simulink model "ibob_phased_array_2k"  (Simulink 7.1)
settings: Solver=ode45  StartTime=0.0  StopTime=70  RelTol=1e-3
undefined symbols (not defined in the file or in its folder): iBOB
libraries: xbsIndex_r4 x1407, xps_library x46, cfa_library x16, casper_library_sources x8, casper_library_misc x4
(part 1 of 18)
settings Model: Creator=Administrator  LastModifiedBy=Rurik A Primiani
settings DebuggingCC: SaveWithParameterizedLinksMsg=none  SignalResolutionControl=TryResolveAllWithWarning  MultiTaskDSMMsg=warning  MultiTaskCondExecSysMsg=none  StrictBusMsg=None
settings RTWCC: IncludeERTFirstTime=on
settings GRTTargetCC: TargetFcnLib=ansi_tfl_tmw.mat

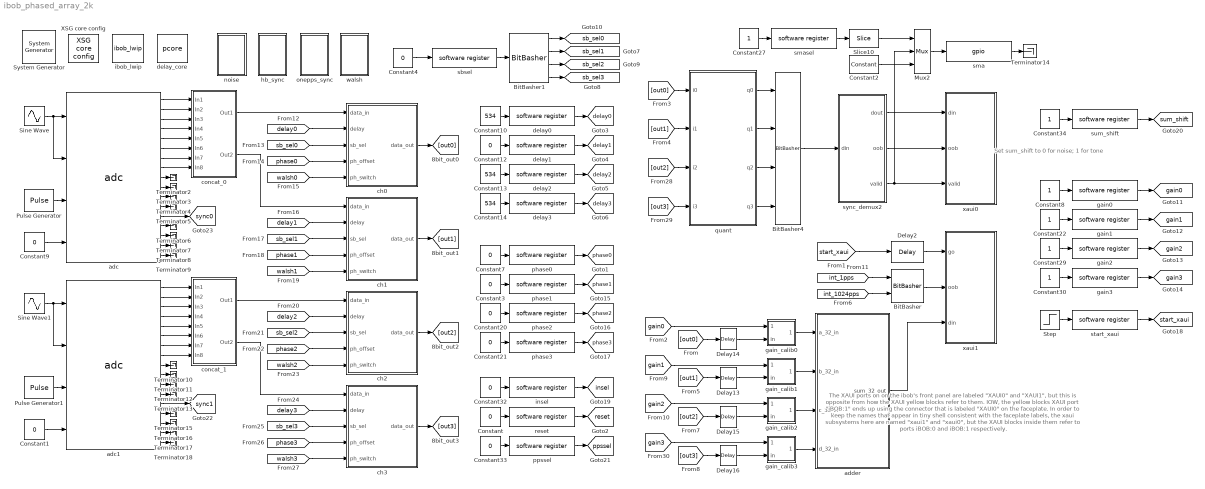
== system ibob_phased_array_2k ==
  note: The XAUI ports on on the ibob's front panel are labeled "XAUI0"
      | and "XAUI1", but this is opposite from how the XAUI yellow blocks
      | refer to them.  IOW, the yellow blocks XAUI port "iBOB:1" ends up
      | using the connector that is labeled "XAUI0" on the faceplate.
      |
      | In order to keep the names that appear in tiny shell consistent with
      | the faceplate labels, the xaui subsystems here are named "xaui1"
      | and "xaui0", but the XAUI blocks inside them refer to ports iBOB:0
      | and iBOB:1 respectively.
  note: Set sum_shift to 0 for noise; 1 for tone
  " System Generator" : xbsIndex_r4/ System Generator  Tag=genX  SystemSampleTime=-1  xilinxfamily=virtex2p  part=xc2vp50  speed=-7  package=ff1152  synthesis_tool=XST  clock_wrapper=Clock Enables  directory=./ibob_phased_array_2k/sysgen  testbench=off  simulink_period=1  sysclk_period=3.9063  dcm_input_clock_period=100  incr_netlist=off  trim_vbits=Everywhere in SubSystem  dbl_ovrd=According to Block Masks  core_generation=According to Block Masks  run_coregen=off  deprecated_control=off  eval_field=0  block_type=sysgen
      settings: block_version=10.1.3
  BitBasher : xbsIndex_r4/BitBasher  bitexpr=|  display_expr=off  sr_1=1  arith_type1=Unsigned  bin_pt1=0  sr_2=2  arith_type2=Unsigned  bin_pt2=0  sr_3=3  arith_type3=Unsigned  bin_pt3=0  sr_4=4  arith_type4=Unsigned  bin_pt4=0  dbl_ovrd=off  block_type=bitbasher
      | <html><head><meta name="qrichtext" content="1" /><style type="text/css">
      | p, li { white-space: pre-wrap; }
      | </style></head><body style=" font-family:'MS Shell Dlg 2'; font-size:8.25pt; font-weight:400; font-style:normal;">
      | <p style=" margin-top:12px; margin-bottom:12px; margin-left:0px; margin-right:0px; -qt-block-indent:0; text-indent:0px; font-family:'MS Shell Dlg'; font-size:8pt;">oob={2'b00,pps1,pps1024}</p></body></html>
      settings: block_version=10.1.3
  BitBasher1 : xbsIndex_r4/BitBasher  bitexpr=|  display_expr=off  sr_1=1  arith_type1=Unsigned  bin_pt1=0  sr_2=2  arith_type2=Unsigned  bin_pt2=0  sr_3=3  arith_type3=Unsigned  bin_pt3=0  sr_4=4  arith_type4=Unsigned  bin_pt4=0  dbl_ovrd=off  block_type=bitbasher
      | <html><head><meta name="qrichtext" content="1" /><style type="text/css">
      | p, li { white-space: pre-wrap; }
      | </style></head><body style=" font-family:'MS Shell Dlg 2'; font-size:8.25pt; font-weight:400; font-style:normal;">
      | <p style=" margin-top:12px; margin-bottom:12px; margin-left:0px; margin-right:0px; -qt-block-indent:0; text-indent:0px; font-family:'MS Shell Dlg'; font-size:8pt;">sel0={sel[0]}<br />sel1={sel[4]}<br />sel2={sel[8]}<br />sel3={sel[12]}<br /></p></body></html>
      settings: block_version=10.1.3
  BitBasher4 : xbsIndex_r4/BitBasher  bitexpr=|  display_expr=off  sr_1=1  arith_type1=Unsigned  bin_pt1=0  sr_2=2  arith_type2="Signed  (2's comp)"  bin_pt2=7  sr_3=3  arith_type3="Signed  (2's comp)"  bin_pt3=7  sr_4=4  arith_type4="Signed  (2's comp)"  bin_pt4=7  dbl_ovrd=off  block_type=bitbasher
      | <html><head><meta name="qrichtext" content="1" /><style type="text/css">
      | p, li { white-space: pre-wrap; }
      | </style></head><body style=" font-family:'MS Shell Dlg 2'; font-size:8.25pt; font-weight:400; font-style:normal;">
      | <p style=" margin-top:0px; margin-bottom:0px; margin-left:0px; margin-right:0px; -qt-block-indent:0; text-indent:0px; font-size:8pt;">out={in0,in1,in2,in3}</p></body></html>
      settings: block_version=10.1.3
  Constant{,1,3..4,7,9,12,20..21,32..33} (11 alike) : Constant  Value=0  OutDataType=sfix(16)  OutScaling=2^0
  Constant10 : Constant  Value=534  OutDataType=sfix(16)  OutScaling=2^0
  Constant13 : Constant  Value=534  OutDataType=sfix(16)  OutScaling=2^0
  Constant14 : Constant  Value=534  OutDataType=sfix(16)  OutScaling=2^0
  Constant2 : xbsIndex_r4/Constant  arith_type=Boolean  const=0  n_bits=16  bin_pt=14  explicit_period=off  period=1  equ=P=C  opselect=C  inp2=PCIN>>17  opr=+  inp1=P  carry=CIN  dbl_ovrd=off  block_type=constant
  Constant{8,22,27,29..30,34} (6 alike) : Constant  OutDataType=sfix(16)  OutScaling=2^0
  Delay{2,13..16} (5 alike) : xbsIndex_r4/Delay  en=off  latency=10  dbl_ovrd=off  reg_retiming=on  block_type=delay
      settings: xl_area=[0, 0, 0, 0, 0, 0, 0]
  Mux2 : xbsIndex_r4/Mux  inputs=2  en=off  latency=2  precision=Full  arith_type="Signed  (2's comp)"  n_bits=8  bin_pt=2  quantization=Truncate  overflow=Wrap  dbl_ovrd=off  block_type=mux
      settings: xl_area=[0, 0, 0, 0, 0, 0, 0]
  Pulse Generator : DiscretePulseGenerator  Period=100  PulseWidth=20
  Pulse Generator1 : DiscretePulseGenerator  Period=100  PulseWidth=20
  Sine Wave : Sin  SineType=Sample based  Amplitude=0.9  Frequency=6.4340e+9  Samples=60  SampleTime=1/4
  Sine Wave1 : Sin  SineType=Sample based  Amplitude=0.9  Frequency=6.4340e+9  Samples=60  SampleTime=1/4
  Slice10 : xbsIndex_r4/Slice  nbits=1  boolean_output=off  mode=Lower Bit Location + Width  bit1=0  base1=MSB of Input  bit0=0  base0=LSB of Input  dbl_ovrd=off  block_type=slice
      settings: infoedit="Extracts a given range of bits from each input sample and presents it at the output.  The output type is ordinarily unsigned with binary point at zero, but can be Boolean when the slice is one bit wide.<P><P>Hardware notes: In hardware this block costs nothing."  block_version=10.1.3
  Step : Step  Time=100  SampleTime=0
  Terminator{2..18} (17 alike) : Terminator
  XSG core config : xps_library/XSG core config  Tag=xps:xsg  SystemSampleTime=-1  hw_sys=iBOB  ibob_linux=off  clk_src=adc0_clk  iBOB_clk_src=adc0_clk  BEE2_ctrl_clk_src=sys_clk  BEE2_usr_clk_src=sys_clk  ROACH_clk_src=sys_clk  CORR_clk_src=sys_clk  gpio_clk_io_group=iBOB:sma  gpio_clk_bit_index=0  clk_rate=256  sample_period=1  synthesis_tool=XST  mpc_type=powerpc405
  adc : xps_library/adc  Tag=xps:adc  SystemSampleTime=-1  adc_brd=adc0  adc_clk_rate=1024  adc_interleave=off  sample_period=1
  adc1 : xps_library/adc  Tag=xps:adc  SystemSampleTime=-1  adc_brd=adc1  adc_clk_rate=1024  adc_interleave=off  sample_period=1
  adder : Subsystem
  ch0 : Subsystem
  ch1 : Subsystem
  ch2 : Subsystem
  ch3 : Subsystem
  concat_0 : Subsystem
  concat_1 : Subsystem
  delay0 : xps_library/software register  Tag=xps:sw_reg  SystemSampleTime=-1  io_dir=From Processor  arith_type=Unsigned  bitwidth=32  bin_pt=0  sample_period=1  gw_name=ibob_phased_array_2k_delay0_user_data_out
      link override ibob_phased_array_2k_delay0_user_data_out: arith_type=Unsigned  n_bits=32  bin_pt=0  period=1
      link override ibob_phased_array_2k_delay1_user_data_out: arith_type=Unsigned  n_bits=32  bin_pt=0  period=1
  delay1 : xps_library/software register  Tag=xps:sw_reg  SystemSampleTime=-1  io_dir=From Processor  arith_type=Unsigned  bitwidth=32  bin_pt=0  sample_period=1  gw_name=ibob_phased_array_2k_delay1_user_data_out
      link override ibob_phased_array_2k_delay1_user_data_out: arith_type=Unsigned  n_bits=32  bin_pt=0  period=1
      link override ibob_phased_array_2k_delay2_user_data_out: arith_type=Unsigned  n_bits=32  bin_pt=0  period=1
  delay2 : xps_library/software register  Tag=xps:sw_reg  SystemSampleTime=-1  io_dir=From Processor  arith_type=Unsigned  bitwidth=32  bin_pt=0  sample_period=1  gw_name=ibob_phased_array_2k_delay2_user_data_out
      link override ibob_phased_array_2k_delay2_user_data_out: arith_type=Unsigned  n_bits=32  bin_pt=0  period=1
      link override ibob_phased_array_2k_delay3_user_data_out: arith_type=Unsigned  n_bits=32  bin_pt=0  period=1
  delay3 : xps_library/software register  Tag=xps:sw_reg  SystemSampleTime=-1  io_dir=From Processor  arith_type=Unsigned  bitwidth=32  bin_pt=0  sample_period=1  gw_name=ibob_phased_array_2k_delay3_user_data_out
      link override ibob_phased_array_2k_delay3_user_data_out: arith_type=Unsigned  n_bits=32  bin_pt=0  period=1
      link override ibob_phased_array_2k_delay4_user_data_out: arith_type=Unsigned  n_bits=32  bin_pt=0  period=1
  delay_core : xps_library/pcore  Tag=xps:pcore  SystemSampleTime=-1  pcore_path=delay_core/delay_core.ngc
  gain0 : xps_library/software register  Tag=xps:sw_reg  SystemSampleTime=-1  io_dir=From Processor  arith_type=Unsigned  bitwidth=32  bin_pt=0  sample_period=1  gw_name=ibob_phased_array_2k_gain0_user_data_out
      link override ibob_phased_array_2k_gain0_user_data_out: arith_type=Unsigned  n_bits=32  bin_pt=0  period=1
  gain1 : xps_library/software register  Tag=xps:sw_reg  SystemSampleTime=-1  io_dir=From Processor  arith_type=Unsigned  bitwidth=32  bin_pt=0  sample_period=1  gw_name=ibob_phased_array_2k_gain1_user_data_out
      link override ibob_phased_array_2k_gain1_user_data_out: arith_type=Unsigned  n_bits=32  bin_pt=0  period=1
  gain2 : xps_library/software register  Tag=xps:sw_reg  SystemSampleTime=-1  io_dir=From Processor  arith_type=Unsigned  bitwidth=32  bin_pt=0  sample_period=1  gw_name=ibob_phased_array_2k_gain2_user_data_out
      link override ibob_phased_array_2k_gain2_user_data_out: arith_type=Unsigned  n_bits=32  bin_pt=0  period=1
  gain3 : xps_library/software register  Tag=xps:sw_reg  SystemSampleTime=-1  io_dir=From Processor  arith_type=Unsigned  bitwidth=32  bin_pt=0  sample_period=1  gw_name=ibob_phased_array_2k_gain3_user_data_out
      link override ibob_phased_array_2k_gain3_user_data_out: arith_type=Unsigned  n_bits=32  bin_pt=0  period=1
  gain_calib0 : Subsystem
  gain_calib1 : Subsystem
  gain_calib2 : Subsystem
  gain_calib3 : Subsystem
  hb_sync : Subsystem
  ibob_lwip : xps_library/ibob_lwip  SystemSampleTime=-1
      link override macbits/convert: arith_type=Unsigned  n_bits=32  bin_pt=0
      link override machdr/ibob_phased_array_2k_ibob_lwip_machdr_gateway: arith_type=Unsigned  n_bits=20  bin_pt=0  period=sample_period
  insel : xps_library/software register  Tag=xps:sw_reg  SystemSampleTime=-1  io_dir=From Processor  arith_type=Unsigned  bitwidth=32  bin_pt=0  sample_period=1  gw_name=ibob_phased_array_2k_insel_user_data_out
      link override ibob_phased_array_2k_insel_user_data_out: arith_type=Unsigned  n_bits=32  bin_pt=0  period=1
      link override ibob_phased_array_2k_reset_user_data_out: arith_type=Unsigned  n_bits=32  bin_pt=0  period=1
  noise : Subsystem
  onepps_sync : Subsystem
  phase0 : xps_library/software register  Tag=xps:sw_reg  SystemSampleTime=-1  io_dir=From Processor  arith_type=Unsigned  bitwidth=32  bin_pt=0  sample_period=1  gw_name=ibob_phased_array_2k_phase0_user_data_out
      link override ibob_phased_array_2k_bypass1_user_data_out: arith_type=Unsigned  n_bits=32  bin_pt=0  period=1
      link override ibob_phased_array_2k_phase0_user_data_out: arith_type=Unsigned  n_bits=32  bin_pt=0  period=1
  phase1 : xps_library/software register  Tag=xps:sw_reg  SystemSampleTime=-1  io_dir=From Processor  arith_type=Unsigned  bitwidth=32  bin_pt=0  sample_period=1  gw_name=ibob_phased_array_2k_phase1_user_data_out
      link override ibob_phased_array_2k_bypass2_user_data_out: arith_type=Unsigned  n_bits=32  bin_pt=0  period=1
      link override ibob_phased_array_2k_phase1_user_data_out: arith_type=Unsigned  n_bits=32  bin_pt=0  period=1
  phase2 : xps_library/software register  Tag=xps:sw_reg  SystemSampleTime=-1  io_dir=From Processor  arith_type=Unsigned  bitwidth=32  bin_pt=0  sample_period=1  gw_name=ibob_phased_array_2k_phase2_user_data_out
      link override ibob_phased_array_2k_bypass3_user_data_out: arith_type=Unsigned  n_bits=32  bin_pt=0  period=1
      link override ibob_phased_array_2k_phase2_user_data_out: arith_type=Unsigned  n_bits=32  bin_pt=0  period=1
  phase3 : xps_library/software register  Tag=xps:sw_reg  SystemSampleTime=-1  io_dir=From Processor  arith_type=Unsigned  bitwidth=32  bin_pt=0  sample_period=1  gw_name=ibob_phased_array_2k_phase3_user_data_out
      link override ibob_phased_array_2k_bypass4_user_data_out: arith_type=Unsigned  n_bits=32  bin_pt=0  period=1
      link override ibob_phased_array_2k_phase3_user_data_out: arith_type=Unsigned  n_bits=32  bin_pt=0  period=1
  ppssel : xps_library/software register  Tag=xps:sw_reg  SystemSampleTime=-1  io_dir=From Processor  arith_type=Unsigned  bitwidth=32  bin_pt=0  sample_period=1  gw_name=ibob_phased_array_2k_ppssel_user_data_out
      link override ibob_phased_array_2k_ppssel_user_data_out: arith_type=Unsigned  n_bits=32  bin_pt=0  period=1
      link override ibob_phased_array_2k_reset_user_data_out: arith_type=Unsigned  n_bits=32  bin_pt=0  period=1
  quant : Subsystem
  reset : xps_library/software register  Tag=xps:sw_reg  SystemSampleTime=-1  io_dir=From Processor  arith_type=Unsigned  bitwidth=32  bin_pt=0  sample_period=1  gw_name=ibob_phased_array_2k_reset_user_data_out
      link override ibob_phased_array_2k_reset_user_data_out: arith_type=Unsigned  n_bits=32  bin_pt=0  period=1
  sbsel : xps_library/software register  Tag=xps:sw_reg  SystemSampleTime=-1  io_dir=From Processor  arith_type=Unsigned  bitwidth=32  bin_pt=0  sample_period=1  gw_name=ibob_phased_array_2k_sbsel_user_data_out
      link override dbe_adc_single_noise_arm_user_data_out: arith_type=Unsigned  n_bits=32  bin_pt=0  period=1
      link override dbe_adc_single_shiftctrl_reg_user_data_out: arith_type=Unsigned  n_bits=32  bin_pt=0  period=1
      link override ibob_phased_array_2k_noise_arm_user_data_out: arith_type=Unsigned  n_bits=32  bin_pt=0  period=1
      link override ibob_phased_array_2k_sb_sel_user_data_out: arith_type=Unsigned  n_bits=32  bin_pt=0  period=1
      link override ibob_phased_array_2k_sbsel_user_data_out: arith_type=Unsigned  n_bits=32  bin_pt=0  period=1
      link override vlbipfb2_m3_ibob_shiftctrl_reg_user_data_out: arith_type=Unsigned  n_bits=32  bin_pt=0  period=1
      link override vlbipfb2_m3_roach_shiftctrl_reg_user_data_out: arith_type=Unsigned  n_bits=32  bin_pt=0  period=1
  sma : xps_library/gpio  Tag=xps:gpio  SystemSampleTime=-1  io_group=iBOB:sma  io_dir=out  arith_type=Boolean  bitwidth=1  bin_pt=0  bit_index=1  sample_period=1  use_single_ended=off  use_ddr=off  reg_iob=on  reg_clk_phase=0  termination=None
      link override convert: arith_type=Boolean  n_bits=1  bin_pt=0
  smasel : xps_library/software register  Tag=xps:sw_reg  SystemSampleTime=-1  io_dir=From Processor  arith_type=Unsigned  bitwidth=32  bin_pt=0  sample_period=1  gw_name=ibob_phased_array_2k_smasel_user_data_out
      link override ibob_phased_array_2k_smasel_user_data_out: arith_type=Unsigned  n_bits=32  bin_pt=0  period=1
  start_xaui : xps_library/software register  Tag=xps:sw_reg  SystemSampleTime=-1  io_dir=From Processor  arith_type=Unsigned  bitwidth=32  bin_pt=0  sample_period=1  gw_name=ibob_phased_array_2k_start_xaui_user_data_out
      link override ibob_phased_array_2k_start_xaui_user_data_out: arith_type=Unsigned  n_bits=32  bin_pt=0  period=1
  sum_shift : xps_library/software register  Tag=xps:sw_reg  SystemSampleTime=-1  io_dir=From Processor  arith_type=Unsigned  bitwidth=32  bin_pt=0  sample_period=1  gw_name=ibob_phased_array_2k_sum_shift_user_data_out
      link override ibob_phased_array_2k_gain0_user_data_out: arith_type=Unsigned  n_bits=32  bin_pt=0  period=1
      link override ibob_phased_array_2k_sum_shift_user_data_out: arith_type=Unsigned  n_bits=32  bin_pt=0  period=1
  sync_demux2 : Subsystem  mask{walsh_delay=5, phsw_delay=21, quant_delay=4}
      mask prompts: walsh_delay "Walsh Latency:"; phsw_delay "Phase Swith Latency:"; quant_delay "Quantizer Latency:"
      mask help: Please enter the appropriate delay values to align the phase switching signals to the data.
  walsh : Subsystem
  xaui0 : Subsystem
  xaui1 : Subsystem
  tag scope: delay0=global, delay1=global, delay2=global, delay3=global, gain0=global, gain1=global, gain2=global, gain3=global, insel=global, phase0=global, phase1=global, phase2=global, phase3=global, ppssel=global, reset=global, sb_sel0=global, sb_sel1=global, sb_sel2=global, sb_sel3=global, start_xaui=global, sum_shift=global, sync0=global, sync1=global
  wires:
  Constant9/1 -> adc/4
  Constant1/1 -> adc1/4
  Constant/1 -> reset/1
  Constant12/1 -> delay1/1
  Constant13/1 -> delay2/1
  Constant14/1 -> delay3/1
  reset/1 -> [reset]
  delay1/1 -> [delay1]
  delay2/1 -> [delay2]
  delay3/1 -> [delay3]
  Sine Wave1/1 -> adc1/1, adc1/2
  Sine Wave/1 -> adc/1, adc/2
  Constant10/1 -> delay0/1
  delay0/1 -> [delay0]
  Pulse Generator/1 -> adc/3
  Pulse Generator1/1 -> adc1/3
  sync_demux2/3(valid) -> xaui0/3(valid), Mux2/2
  adc/13 -> [sync0]
  sma/1 -> Terminator14/1
  adc/1 -> concat_0/1(In1)
  adc/2 -> concat_0/2(In2)
  adc/3 -> concat_0/3(In3)
  adc/4 -> concat_0/4(In4)
  adc/5 -> concat_0/5(In5)
  adc/6 -> concat_0/6(In6)
  adc/7 -> concat_0/7(In7)
  adc/8 -> concat_0/8(In8)
  adc1/1 -> concat_1/1(In1)
  adc1/2 -> concat_1/2(In2)
  adc1/3 -> concat_1/3(In3)
  adc1/4 -> concat_1/4(In4)
  adc1/5 -> concat_1/5(In5)
  adc1/6 -> concat_1/6(In6)
  adc1/7 -> concat_1/7(In7)
  adc1/8 -> concat_1/8(In8)
  sync_demux2/2(oob) -> xaui0/2(oob)
  Mux2/1 -> sma/1
  smasel/1 -> Slice10/1
  Constant27/1 -> smasel/1
  Slice10/1 -> Mux2/1
  adder/1(sum_32_out) -> xaui1/3(din)
  [start_xaui] -> Delay2/1
  BitBasher/1 -> xaui1/2(oob)
  [gain0] -> gain_calib0/1(gain)
  [gain1] -> gain_calib1/1(gain)
  [gain2] -> gain_calib2/1(gain)
  [gain3] -> gain_calib3/1(gain)
  gain_calib0/1(out) -> adder/1(a_32_in)
  gain_calib1/1(out) -> adder/2(b_32_in)
  gain_calib2/1(out) -> adder/3(c_32_in)
  gain_calib3/1(out) -> adder/4(d_32_in)
  [out0] -> Delay14/1
  [out1] -> Delay13/1
  [out2] -> Delay15/1
  [out3] -> Delay16/1
  sync_demux2/1(dout) -> xaui0/1(din)
  Delay14/1 -> gain_calib0/2(in)
  Delay13/1 -> gain_calib1/2(in)
  Delay15/1 -> gain_calib2/2(in)
  Delay16/1 -> gain_calib3/2(in)
  Constant32/1 -> insel/1
  insel/1 -> [insel]
  Constant33/1 -> ppssel/1
  ppssel/1 -> [ppssel]
  adc1/13 -> [sync1]
  Constant34/1 -> sum_shift/1
  sum_shift/1 -> [sum_shift]
  [int_1024pps] -> BitBasher/2
  [int_1pps] -> BitBasher/1
  sbsel/1 -> BitBasher1/1
  Constant4/1 -> sbsel/1
  BitBasher1/1 -> [sb_sel0]
  BitBasher1/2 -> [sb_sel1]
  BitBasher1/3 -> [sb_sel2]
  BitBasher1/4 -> [sb_sel3]
  Constant7/1 -> phase0/1
  phase0/1 -> [phase0]
  Constant3/1 -> phase1/1
  phase1/1 -> [phase1]
  Constant20/1 -> phase2/1
  phase2/1 -> [phase2]
  Constant21/1 -> phase3/1
  phase3/1 -> [phase3]
  concat_0/1(Out1) -> ch0/1(data_in)
  [delay0] -> ch0/2(delay)
  [sb_sel0] -> ch0/3(sb_sel)
  [phase0] -> ch0/4(ph_offset)
  [walsh0] -> ch0/5(ph_switch)
  concat_0/2(Out2) -> ch1/1(data_in)
  concat_1/1(Out1) -> ch2/1(data_in)
  concat_1/2(Out2) -> ch3/1(data_in)
  [delay1] -> ch1/2(delay)
  [sb_sel1] -> ch1/3(sb_sel)
  [phase1] -> ch1/4(ph_offset)
  [walsh1] -> ch1/5(ph_switch)
  [delay2] -> ch2/2(delay)
  [sb_sel2] -> ch2/3(sb_sel)
  [phase2] -> ch2/4(ph_offset)
  [walsh2] -> ch2/5(ph_switch)
  [delay3] -> ch3/2(delay)
  [sb_sel3] -> ch3/3(sb_sel)
  [phase3] -> ch3/4(ph_offset)
  [walsh3] -> ch3/5(ph_switch)
  adc/9 -> Terminator2/1
  adc/10 -> Terminator3/1
  adc/11 -> Terminator4/1
  adc/12 -> Terminator5/1
  adc/14 -> Terminator6/1
  adc/15 -> Terminator7/1
  adc/16 -> Terminator8/1
  adc/17 -> Terminator9/1
  adc1/9 -> Terminator10/1
  adc1/10 -> Terminator11/1
  adc1/11 -> Terminator12/1
  adc1/12 -> Terminator13/1
  adc1/14 -> Terminator15/1
  adc1/15 -> Terminator16/1
  adc1/16 -> Terminator17/1
  adc1/17 -> Terminator18/1
  ch0/1(data_out) -> [out0]
  ch1/1(data_out) -> [out1]
  ch2/1(data_out) -> [out2]
  ch3/1(data_out) -> [out3]
  [out0] -> quant/1(i0)
  [out1] -> quant/2(i1)
  [out2] -> quant/3(i2)
  [out3] -> quant/4(i3)
  quant/1(q0) -> BitBasher4/1
  quant/2(q1) -> BitBasher4/2
  quant/3(q2) -> BitBasher4/3
  quant/4(q3) -> BitBasher4/4
  BitBasher4/1 -> sync_demux2/1(din)
  Step/1 -> start_xaui/1
  start_xaui/1 -> [start_xaui]
  Constant2/1 -> Mux2/3
  Constant8/1 -> gain0/1
  Constant22/1 -> gain1/1
  Constant29/1 -> gain2/1
  Constant30/1 -> gain3/1
  gain0/1 -> [gain0]
  gain1/1 -> [gain1]
  gain2/1 -> [gain2]
  gain3/1 -> [gain3]
  Delay2/1 -> xaui1/1(go)

== system ibob_phased_array_2k/adder ==
  a_32_in : Inport  OutDataType=sfix(16)  OutScaling=2^0
  b_32_in : Inport  Port=2  OutDataType=sfix(16)  OutScaling=2^0
  c_32_in : Inport  Port=3  OutDataType=sfix(16)  OutScaling=2^0
  d_32_in : Inport  Port=4  OutDataType=sfix(16)  OutScaling=2^0
  Subsystem : Subsystem
  Subsystem1 : Subsystem
  Subsystem2 : Subsystem
  sum_32_out : Outport  OutDataType=sfix(16)  OutScaling=2^0
  wires:
  Subsystem1/1(Out1) -> Subsystem2/2(b_36_in)
  Subsystem/1(Out1) -> Subsystem2/1(a_36_in)
  d_32_in/1 -> Subsystem1/2(b_32_in)
  c_32_in/1 -> Subsystem1/1(a_32_in)
  b_32_in/1 -> Subsystem/2(b_32_in)
  a_32_in/1 -> Subsystem/1(a_32_in)
  Subsystem2/1(Out1) -> sum_32_out/1

== system ibob_phased_array_2k/ch0 ==
  note: ph_switch and ph_offset take 21 cycles to appear at output
  data_in : Inport  OutDataType=sfix(16)  OutScaling=2^0
  delay : Inport  Port=2  OutDataType=sfix(16)  OutScaling=2^0
  sb_sel : Inport  Port=3  OutDataType=sfix(16)  OutScaling=2^0
  ph_offset : Inport  Port=4  OutDataType=sfix(16)  OutScaling=2^0
  ph_switch : Inport  Port=5  OutDataType=sfix(16)  OutScaling=2^0
  AddSub : xbsIndex_r4/AddSub  mode=Subtraction  use_carryin=off  use_carryout=off  en=off  latency=1  precision=User Defined  arith_type=Unsigned  n_bits=2  bin_pt=0  quantization=Truncate  overflow=Wrap  dbl_ovrd=off  use_behavioral_HDL=off  pipelined=off  use_rpm=on  hw_selection=Fabric  block_type=addsub
      settings: block_version=10.1.3
  AddSub1 : xbsIndex_r4/AddSub  mode=Addition  use_carryin=off  use_carryout=off  en=off  latency=1  precision=User Defined  arith_type=Unsigned  n_bits=2  bin_pt=0  quantization=Truncate  overflow=Wrap  dbl_ovrd=off  use_behavioral_HDL=off  pipelined=off  use_rpm=on  hw_selection=Fabric  block_type=addsub
      settings: block_version=10.1.3
  BitBasher : xbsIndex_r4/BitBasher  bitexpr=|  display_expr=off  sr_1=1  arith_type1="Signed  (2's comp)"  bin_pt1=7  sr_2=2  arith_type2="Signed  (2's comp)"  bin_pt2=7  sr_3=3  arith_type3="Signed  (2's comp)"  bin_pt3=7  sr_4=4  arith_type4="Signed  (2's comp)"  bin_pt4=7  dbl_ovrd=off  block_type=bitbasher
      | <html><head><meta name="qrichtext" content="1" /><style type="text/css">
      | p, li { white-space: pre-wrap; }
      | </style></head><body style=" font-family:'MS Shell Dlg 2'; font-size:8.25pt; font-weight:400; font-style:normal;">
      | <p style=" margin-top:0px; margin-bottom:0px; margin-left:0px; margin-right:0px; -qt-block-indent:0; text-indent:0px;">in0={in[31:24]}<br />in1={in[23:16]}<br />in2={in[15:8]}<br />in3={in[7:0]}<br /></p></body></html>
      settings: block_version=10.1.3
  BitBasher1 : xbsIndex_r4/BitBasher  bitexpr=|  display_expr=off  sr_1=1  arith_type1=Unsigned  bin_pt1=0  sr_2=2  arith_type2=Unsigned  bin_pt2=0  sr_3=3  arith_type3="Signed  (2's comp)"  bin_pt3=7  sr_4=4  arith_type4="Signed  (2's comp)"  bin_pt4=7  dbl_ovrd=off  block_type=bitbasher
      | <html><head><meta name="qrichtext" content="1" /><style type="text/css">
      | p, li { white-space: pre-wrap; }
      | </style></head><body style=" font-family:'MS Shell Dlg 2'; font-size:8.25pt; font-weight:400; font-style:normal;">
      | <p style=" margin-top:0px; margin-bottom:0px; margin-left:0px; margin-right:0px; -qt-block-indent:0; text-indent:0px; font-size:8pt;">div90={phase[11:10]}<br />mod90={phase[9:0]}</p></body></html>
      settings: block_version=10.1.3
  BitBasher2 : xbsIndex_r4/BitBasher  bitexpr=|  display_expr=off  sr_1=1  arith_type1=Unsigned  bin_pt1=0  sr_2=2  arith_type2="Signed  (2's comp)"  bin_pt2=7  sr_3=3  arith_type3="Signed  (2's comp)"  bin_pt3=7  sr_4=4  arith_type4="Signed  (2's comp)"  bin_pt4=7  dbl_ovrd=off  block_type=bitbasher
      | <html><head><meta name="qrichtext" content="1" /><style type="text/css">
      | p, li { white-space: pre-wrap; }
      | </style></head><body style=" font-family:'MS Shell Dlg 2'; font-size:8.25pt; font-weight:400; font-style:normal;">
      | <p style=" margin-top:0px; margin-bottom:0px; margin-left:0px; margin-right:0px; -qt-block-indent:0; text-indent:0px; font-size:8pt;">phase={div90,mod90}</p></body></html>
      settings: block_version=10.1.3
  BitBasher3 : xbsIndex_r4/BitBasher  bitexpr=|  display_expr=off  sr_1=1  arith_type1=Unsigned  bin_pt1=0  sr_2=2  arith_type2="Signed  (2's comp)"  bin_pt2=7  sr_3=3  arith_type3="Signed  (2's comp)"  bin_pt3=7  sr_4=4  arith_type4="Signed  (2's comp)"  bin_pt4=7  dbl_ovrd=off  block_type=bitbasher
      | <html><head><meta name="qrichtext" content="1" /><style type="text/css">
      | p, li { white-space: pre-wrap; }
      | </style></head><body style=" font-family:'MS Shell Dlg 2'; font-size:8.25pt; font-weight:400; font-style:normal;">
      | <p style=" margin-top:0px; margin-bottom:0px; margin-left:0px; margin-right:0px; -qt-block-indent:0; text-indent:0px; font-size:8pt;">out={in0,in1,in2,in3}</p></body></html>
      settings: block_version=10.1.3
  BitBasher4 : xbsIndex_r4/BitBasher  bitexpr=|  display_expr=off  sr_1=1  arith_type1=Unsigned  bin_pt1=4  sr_2=2  arith_type2=Unsigned  bin_pt2=0  sr_3=3  arith_type3="Signed  (2's comp)"  bin_pt3=7  sr_4=4  arith_type4="Signed  (2's comp)"  bin_pt4=7  dbl_ovrd=off  block_type=bitbasher
      | <html><head><meta name="qrichtext" content="1" /><style type="text/css">
      | p, li { white-space: pre-wrap; }
      | </style></head><body style=" font-family:'MS Shell Dlg 2'; font-size:8.25pt; font-weight:400; font-style:normal;">
      | <p style=" margin-top:0px; margin-bottom:0px; margin-left:0px; margin-right:0px; -qt-block-indent:0; text-indent:0px; font-size:8pt;">o={i[16:0]}</p></body></html>
      settings: block_version=10.1.3
  Delay1 : xbsIndex_r4/Delay  en=off  latency=2  dbl_ovrd=off  reg_retiming=off  block_type=delay
  Register{,1..7} (8 alike) : xbsIndex_r4/Register  init=0  rst=off  en=off  dbl_ovrd=off  block_type=register
  SineCosine : xbsIndex_r4/SineCosine  mode=Sine and Cosine  neg_sin=off  neg_cos=off  n_bits=18  sym_output=on  en=off  latency=10  dbl_ovrd=off  explicit_period=off  period=1  mem_type=Block RAM  pipeline=on  use_rpm=off  block_type=sincos
      settings: AttributesFormatString=latency = %<latency>  xl_area=[44 42 1 81 0 0 0]  block_version=10.1.3
  delay_core : xbsIndex_r4/Black Box  init_code=delay_core_config  sim_method=Inactive  block_type=blackbox2
      settings: infoedit="Incorporates black box HDL and simulation model into a System Generator design.<P><P>You must supply a Black Box with certain information about the HDL component you would like to bring into System Generator. This information is provided through a Matlab function.<P><P>When \"Simulation mode\" is set to \"Inactive\", you will typically want to provide a separate simulation model by using a Simulation Multiplexer.<P>When \"Simulation mode\" is set to \"External co-simulator\", you must include a ModelSim block in the design."  block_version=10.1.3
  phase_rotate : Subsystem
      settings: AttributesFormatString=latency=9
  data_out : Outport  OutDataType=sfix(16)  OutScaling=2^0
  wires:
  BitBasher3/1 -> data_out/1
  phase_rotate/4(im2_out) -> BitBasher3/4
  phase_rotate/3(re2_out) -> BitBasher3/3
  phase_rotate/2(im0_out) -> BitBasher3/2
  phase_rotate/1(re0_out) -> BitBasher3/1
  AddSub1/1 -> BitBasher2/1
  AddSub/1 -> AddSub1/2
  delay_core/5 -> AddSub1/1
  SineCosine/2 -> phase_rotate/6(cos)
  SineCosine/1 -> phase_rotate/5(sin)
  data_in/1 -> BitBasher/1
  sb_sel/1 -> delay_core/6
  delay/1 -> BitBasher4/1
  delay_core/4 -> Register3/1
  delay_core/3 -> Register2/1
  delay_core/2 -> Register1/1
  delay_core/1 -> Register/1
  Delay1/1 -> BitBasher2/2
  BitBasher2/1 -> SineCosine/1
  BitBasher1/2 -> Delay1/1
  ph_offset/1 -> BitBasher1/1
  BitBasher/4 -> delay_core/4
  BitBasher/3 -> delay_core/3
  BitBasher/2 -> delay_core/2
  BitBasher/1 -> delay_core/1
  BitBasher4/1 -> delay_core/5
  Register/1 -> Register4/1
  Register1/1 -> Register5/1
  Register2/1 -> Register6/1
  Register3/1 -> Register7/1
  Register4/1 -> phase_rotate/1(re0_in)
  Register5/1 -> phase_rotate/2(im0_in)
  Register6/1 -> phase_rotate/3(re2_in)
  Register7/1 -> phase_rotate/4(im2_in)
  BitBasher1/1 -> AddSub/1
  ph_switch/1 -> AddSub/2

== system ibob_phased_array_2k/ch1 ==
  data_in : Inport  OutDataType=sfix(16)  OutScaling=2^0
  delay : Inport  Port=2  OutDataType=sfix(16)  OutScaling=2^0
  sb_sel : Inport  Port=3  OutDataType=sfix(16)  OutScaling=2^0
  ph_offset : Inport  Port=4  OutDataType=sfix(16)  OutScaling=2^0
  ph_switch : Inport  Port=5  OutDataType=sfix(16)  OutScaling=2^0
  AddSub : xbsIndex_r4/AddSub  mode=Subtraction  use_carryin=off  use_carryout=off  en=off  latency=1  precision=User Defined  arith_type=Unsigned  n_bits=2  bin_pt=0  quantization=Truncate  overflow=Wrap  dbl_ovrd=off  use_behavioral_HDL=off  pipelined=off  use_rpm=on  hw_selection=Fabric  block_type=addsub
      settings: block_version=10.1.3
  AddSub1 : xbsIndex_r4/AddSub  mode=Addition  use_carryin=off  use_carryout=off  en=off  latency=1  precision=User Defined  arith_type=Unsigned  n_bits=2  bin_pt=0  quantization=Truncate  overflow=Wrap  dbl_ovrd=off  use_behavioral_HDL=off  pipelined=off  use_rpm=on  hw_selection=Fabric  block_type=addsub
      settings: block_version=10.1.3
  BitBasher : xbsIndex_r4/BitBasher  bitexpr=|  display_expr=off  sr_1=1  arith_type1="Signed  (2's comp)"  bin_pt1=7  sr_2=2  arith_type2="Signed  (2's comp)"  bin_pt2=7  sr_3=3  arith_type3="Signed  (2's comp)"  bin_pt3=7  sr_4=4  arith_type4="Signed  (2's comp)"  bin_pt4=7  dbl_ovrd=off  block_type=bitbasher
      | <html><head><meta name="qrichtext" content="1" /><style type="text/css">
      | p, li { white-space: pre-wrap; }
      | </style></head><body style=" font-family:'MS Shell Dlg 2'; font-size:8.25pt; font-weight:400; font-style:normal;">
      | <p style=" margin-top:0px; margin-bottom:0px; margin-left:0px; margin-right:0px; -qt-block-indent:0; text-indent:0px;">in0={in[31:24]}<br />in1={in[23:16]}<br />in2={in[15:8]}<br />in3={in[7:0]}<br /></p></body></html>
      settings: block_version=10.1.3
  BitBasher1 : xbsIndex_r4/BitBasher  bitexpr=|  display_expr=off  sr_1=1  arith_type1=Unsigned  bin_pt1=0  sr_2=2  arith_type2=Unsigned  bin_pt2=0  sr_3=3  arith_type3="Signed  (2's comp)"  bin_pt3=7  sr_4=4  arith_type4="Signed  (2's comp)"  bin_pt4=7  dbl_ovrd=off  block_type=bitbasher
      | <html><head><meta name="qrichtext" content="1" /><style type="text/css">
      | p, li { white-space: pre-wrap; }
      | </style></head><body style=" font-family:'MS Shell Dlg 2'; font-size:8.25pt; font-weight:400; font-style:normal;">
      | <p style=" margin-top:0px; margin-bottom:0px; margin-left:0px; margin-right:0px; -qt-block-indent:0; text-indent:0px; font-size:8pt;">div90={phase[11:10]}<br />mod90={phase[9:0]}</p></body></html>
      settings: block_version=10.1.3
  BitBasher2 : xbsIndex_r4/BitBasher  bitexpr=|  display_expr=off  sr_1=1  arith_type1=Unsigned  bin_pt1=0  sr_2=2  arith_type2="Signed  (2's comp)"  bin_pt2=7  sr_3=3  arith_type3="Signed  (2's comp)"  bin_pt3=7  sr_4=4  arith_type4="Signed  (2's comp)"  bin_pt4=7  dbl_ovrd=off  block_type=bitbasher
      | <html><head><meta name="qrichtext" content="1" /><style type="text/css">
      | p, li { white-space: pre-wrap; }
      | </style></head><body style=" font-family:'MS Shell Dlg 2'; font-size:8.25pt; font-weight:400; font-style:normal;">
      | <p style=" margin-top:0px; margin-bottom:0px; margin-left:0px; margin-right:0px; -qt-block-indent:0; text-indent:0px; font-size:8pt;">phase={div90,mod90}</p></body></html>
      settings: block_version=10.1.3
  BitBasher3 : xbsIndex_r4/BitBasher  bitexpr=|  display_expr=off  sr_1=1  arith_type1=Unsigned  bin_pt1=0  sr_2=2  arith_type2="Signed  (2's comp)"  bin_pt2=7  sr_3=3  arith_type3="Signed  (2's comp)"  bin_pt3=7  sr_4=4  arith_type4="Signed  (2's comp)"  bin_pt4=7  dbl_ovrd=off  block_type=bitbasher
      | <html><head><meta name="qrichtext" content="1" /><style type="text/css">
      | p, li { white-space: pre-wrap; }
      | </style></head><body style=" font-family:'MS Shell Dlg 2'; font-size:8.25pt; font-weight:400; font-style:normal;">
      | <p style=" margin-top:0px; margin-bottom:0px; margin-left:0px; margin-right:0px; -qt-block-indent:0; text-indent:0px; font-size:8pt;">out={in0,in1,in2,in3}</p></body></html>
      settings: block_version=10.1.3
  BitBasher4 : xbsIndex_r4/BitBasher  bitexpr=|  display_expr=off  sr_1=1  arith_type1=Unsigned  bin_pt1=4  sr_2=2  arith_type2=Unsigned  bin_pt2=0  sr_3=3  arith_type3="Signed  (2's comp)"  bin_pt3=7  sr_4=4  arith_type4="Signed  (2's comp)"  bin_pt4=7  dbl_ovrd=off  block_type=bitbasher
      | <html><head><meta name="qrichtext" content="1" /><style type="text/css">
      | p, li { white-space: pre-wrap; }
      | </style></head><body style=" font-family:'MS Shell Dlg 2'; font-size:8.25pt; font-weight:400; font-style:normal;">
      | <p style=" margin-top:0px; margin-bottom:0px; margin-left:0px; margin-right:0px; -qt-block-indent:0; text-indent:0px; font-size:8pt;">o={i[16:0]}</p></body></html>
      settings: block_version=10.1.3
  Delay1 : xbsIndex_r4/Delay  en=off  latency=2  dbl_ovrd=off  reg_retiming=off  block_type=delay
  Register{,1..7} (8 alike) : xbsIndex_r4/Register  init=0  rst=off  en=off  dbl_ovrd=off  block_type=register
  SineCosine : xbsIndex_r4/SineCosine  mode=Sine and Cosine  neg_sin=off  neg_cos=off  n_bits=18  sym_output=on  en=off  latency=10  dbl_ovrd=off  explicit_period=off  period=1  mem_type=Block RAM  pipeline=on  use_rpm=off  block_type=sincos
      settings: AttributesFormatString=latency = %<latency>  xl_area=[44 42 1 81 0 0 0]  block_version=10.1.3
  delay_core : xbsIndex_r4/Black Box  init_code=delay_core_config  sim_method=Inactive  block_type=blackbox2
      settings: infoedit="Incorporates black box HDL and simulation model into a System Generator design.<P><P>You must supply a Black Box with certain information about the HDL component you would like to bring into System Generator. This information is provided through a Matlab function.<P><P>When \"Simulation mode\" is set to \"Inactive\", you will typically want to provide a separate simulation model by using a Simulation Multiplexer.<P>When \"Simulation mode\" is set to \"External co-simulator\", you must include a ModelSim block in the design."  block_version=10.1.3
  phase_rotate : Subsystem
      settings: AttributesFormatString=latency=7
  data_out : Outport  OutDataType=sfix(16)  OutScaling=2^0
  wires:
  BitBasher3/1 -> data_out/1
  phase_rotate/4(im2_out) -> BitBasher3/4
  phase_rotate/3(re2_out) -> BitBasher3/3
  phase_rotate/2(im0_out) -> BitBasher3/2
  phase_rotate/1(re0_out) -> BitBasher3/1
  AddSub1/1 -> BitBasher2/1
  AddSub/1 -> AddSub1/2
  delay_core/5 -> AddSub1/1
  SineCosine/2 -> phase_rotate/6(cos)
  SineCosine/1 -> phase_rotate/5(sin)
  data_in/1 -> BitBasher/1
  sb_sel/1 -> delay_core/6
  delay/1 -> BitBasher4/1
  delay_core/4 -> Register3/1
  delay_core/3 -> Register2/1
  delay_core/2 -> Register1/1
  delay_core/1 -> Register/1
  Delay1/1 -> BitBasher2/2
  BitBasher2/1 -> SineCosine/1
  BitBasher1/2 -> Delay1/1
  ph_offset/1 -> BitBasher1/1
  BitBasher/4 -> delay_core/4
  BitBasher/3 -> delay_core/3
  BitBasher/2 -> delay_core/2
  BitBasher/1 -> delay_core/1
  BitBasher4/1 -> delay_core/5
  Register/1 -> Register4/1
  Register1/1 -> Register5/1
  Register2/1 -> Register6/1
  Register3/1 -> Register7/1
  Register4/1 -> phase_rotate/1(re0_in)
  Register5/1 -> phase_rotate/2(im0_in)
  Register6/1 -> phase_rotate/3(re2_in)
  Register7/1 -> phase_rotate/4(im2_in)
  BitBasher1/1 -> AddSub/1
  ph_switch/1 -> AddSub/2

== system ibob_phased_array_2k/ch2 ==
  data_in : Inport  OutDataType=sfix(16)  OutScaling=2^0
  delay : Inport  Port=2  OutDataType=sfix(16)  OutScaling=2^0
  sb_sel : Inport  Port=3  OutDataType=sfix(16)  OutScaling=2^0
  ph_offset : Inport  Port=4  OutDataType=sfix(16)  OutScaling=2^0
  ph_switch : Inport  Port=5  OutDataType=sfix(16)  OutScaling=2^0
  AddSub : xbsIndex_r4/AddSub  mode=Subtraction  use_carryin=off  use_carryout=off  en=off  latency=1  precision=User Defined  arith_type=Unsigned  n_bits=2  bin_pt=0  quantization=Truncate  overflow=Wrap  dbl_ovrd=off  use_behavioral_HDL=off  pipelined=off  use_rpm=on  hw_selection=Fabric  block_type=addsub
      settings: block_version=10.1.3
  AddSub1 : xbsIndex_r4/AddSub  mode=Addition  use_carryin=off  use_carryout=off  en=off  latency=1  precision=User Defined  arith_type=Unsigned  n_bits=2  bin_pt=0  quantization=Truncate  overflow=Wrap  dbl_ovrd=off  use_behavioral_HDL=off  pipelined=off  use_rpm=on  hw_selection=Fabric  block_type=addsub
      settings: block_version=10.1.3
  BitBasher : xbsIndex_r4/BitBasher  bitexpr=|  display_expr=off  sr_1=1  arith_type1="Signed  (2's comp)"  bin_pt1=7  sr_2=2  arith_type2="Signed  (2's comp)"  bin_pt2=7  sr_3=3  arith_type3="Signed  (2's comp)"  bin_pt3=7  sr_4=4  arith_type4="Signed  (2's comp)"  bin_pt4=7  dbl_ovrd=off  block_type=bitbasher
      | <html><head><meta name="qrichtext" content="1" /><style type="text/css">
      | p, li { white-space: pre-wrap; }
      | </style></head><body style=" font-family:'MS Shell Dlg 2'; font-size:8.25pt; font-weight:400; font-style:normal;">
      | <p style=" margin-top:0px; margin-bottom:0px; margin-left:0px; margin-right:0px; -qt-block-indent:0; text-indent:0px;">in0={in[31:24]}<br />in1={in[23:16]}<br />in2={in[15:8]}<br />in3={in[7:0]}<br /></p></body></html>
      settings: block_version=10.1.3
  BitBasher1 : xbsIndex_r4/BitBasher  bitexpr=|  display_expr=off  sr_1=1  arith_type1=Unsigned  bin_pt1=0  sr_2=2  arith_type2=Unsigned  bin_pt2=0  sr_3=3  arith_type3="Signed  (2's comp)"  bin_pt3=7  sr_4=4  arith_type4="Signed  (2's comp)"  bin_pt4=7  dbl_ovrd=off  block_type=bitbasher
      | <html><head><meta name="qrichtext" content="1" /><style type="text/css">
      | p, li { white-space: pre-wrap; }
      | </style></head><body style=" font-family:'MS Shell Dlg 2'; font-size:8.25pt; font-weight:400; font-style:normal;">
      | <p style=" margin-top:0px; margin-bottom:0px; margin-left:0px; margin-right:0px; -qt-block-indent:0; text-indent:0px; font-size:8pt;">div90={phase[11:10]}<br />mod90={phase[9:0]}</p></body></html>
      settings: block_version=10.1.3
  BitBasher2 : xbsIndex_r4/BitBasher  bitexpr=|  display_expr=off  sr_1=1  arith_type1=Unsigned  bin_pt1=0  sr_2=2  arith_type2="Signed  (2's comp)"  bin_pt2=7  sr_3=3  arith_type3="Signed  (2's comp)"  bin_pt3=7  sr_4=4  arith_type4="Signed  (2's comp)"  bin_pt4=7  dbl_ovrd=off  block_type=bitbasher
      | <html><head><meta name="qrichtext" content="1" /><style type="text/css">
      | p, li { white-space: pre-wrap; }
      | </style></head><body style=" font-family:'MS Shell Dlg 2'; font-size:8.25pt; font-weight:400; font-style:normal;">
      | <p style=" margin-top:0px; margin-bottom:0px; margin-left:0px; margin-right:0px; -qt-block-indent:0; text-indent:0px; font-size:8pt;">phase={div90,mod90}</p></body></html>
      settings: block_version=10.1.3
  BitBasher3 : xbsIndex_r4/BitBasher  bitexpr=|  display_expr=off  sr_1=1  arith_type1=Unsigned  bin_pt1=0  sr_2=2  arith_type2="Signed  (2's comp)"  bin_pt2=7  sr_3=3  arith_type3="Signed  (2's comp)"  bin_pt3=7  sr_4=4  arith_type4="Signed  (2's comp)"  bin_pt4=7  dbl_ovrd=off  block_type=bitbasher
      | <html><head><meta name="qrichtext" content="1" /><style type="text/css">
      | p, li { white-space: pre-wrap; }
      | </style></head><body style=" font-family:'MS Shell Dlg 2'; font-size:8.25pt; font-weight:400; font-style:normal;">
      | <p style=" margin-top:0px; margin-bottom:0px; margin-left:0px; margin-right:0px; -qt-block-indent:0; text-indent:0px; font-size:8pt;">out={in0,in1,in2,in3}</p></body></html>
      settings: block_version=10.1.3
  BitBasher4 : xbsIndex_r4/BitBasher  bitexpr=|  display_expr=off  sr_1=1  arith_type1=Unsigned  bin_pt1=4  sr_2=2  arith_type2=Unsigned  bin_pt2=0  sr_3=3  arith_type3="Signed  (2's comp)"  bin_pt3=7  sr_4=4  arith_type4="Signed  (2's comp)"  bin_pt4=7  dbl_ovrd=off  block_type=bitbasher
      | <html><head><meta name="qrichtext" content="1" /><style type="text/css">
      | p, li { white-space: pre-wrap; }
      | </style></head><body style=" font-family:'MS Shell Dlg 2'; font-size:8.25pt; font-weight:400; font-style:normal;">
      | <p style=" margin-top:0px; margin-bottom:0px; margin-left:0px; margin-right:0px; -qt-block-indent:0; text-indent:0px; font-size:8pt;">o={i[16:0]}</p></body></html>
      settings: block_version=10.1.3
  Delay1 : xbsIndex_r4/Delay  en=off  latency=2  dbl_ovrd=off  reg_retiming=off  block_type=delay
  Register{,1..7} (8 alike) : xbsIndex_r4/Register  init=0  rst=off  en=off  dbl_ovrd=off  block_type=register
  SineCosine : xbsIndex_r4/SineCosine  mode=Sine and Cosine  neg_sin=off  neg_cos=off  n_bits=18  sym_output=on  en=off  latency=10  dbl_ovrd=off  explicit_period=off  period=1  mem_type=Block RAM  pipeline=on  use_rpm=off  block_type=sincos
      settings: AttributesFormatString=latency = %<latency>  xl_area=[44 42 1 81 0 0 0]  block_version=10.1.3
  delay_core : xbsIndex_r4/Black Box  init_code=delay_core_config  sim_method=Inactive  block_type=blackbox2
      settings: infoedit="Incorporates black box HDL and simulation model into a System Generator design.<P><P>You must supply a Black Box with certain information about the HDL component you would like to bring into System Generator. This information is provided through a Matlab function.<P><P>When \"Simulation mode\" is set to \"Inactive\", you will typically want to provide a separate simulation model by using a Simulation Multiplexer.<P>When \"Simulation mode\" is set to \"External co-simulator\", you must include a ModelSim block in the design."  block_version=10.1.3
  phase_rotate : Subsystem
      settings: AttributesFormatString=latency=7
  data_out : Outport  OutDataType=sfix(16)  OutScaling=2^0
  wires:
  BitBasher3/1 -> data_out/1
  phase_rotate/4(im2_out) -> BitBasher3/4
  phase_rotate/3(re2_out) -> BitBasher3/3
  phase_rotate/2(im0_out) -> BitBasher3/2
  phase_rotate/1(re0_out) -> BitBasher3/1
  AddSub1/1 -> BitBasher2/1
  AddSub/1 -> AddSub1/2
  delay_core/5 -> AddSub1/1
  SineCosine/2 -> phase_rotate/6(cos)
  SineCosine/1 -> phase_rotate/5(sin)
  data_in/1 -> BitBasher/1
  sb_sel/1 -> delay_core/6
  delay/1 -> BitBasher4/1
  delay_core/4 -> Register3/1
  delay_core/3 -> Register2/1
  delay_core/2 -> Register1/1
  delay_core/1 -> Register/1
  Delay1/1 -> BitBasher2/2
  BitBasher2/1 -> SineCosine/1
  BitBasher1/2 -> Delay1/1
  ph_offset/1 -> BitBasher1/1
  BitBasher/4 -> delay_core/4
  BitBasher/3 -> delay_core/3
  BitBasher/2 -> delay_core/2
  BitBasher/1 -> delay_core/1
  BitBasher4/1 -> delay_core/5
  Register/1 -> Register4/1
  Register1/1 -> Register5/1
  Register2/1 -> Register6/1
  Register3/1 -> Register7/1
  Register4/1 -> phase_rotate/1(re0_in)
  Register5/1 -> phase_rotate/2(im0_in)
  Register6/1 -> phase_rotate/3(re2_in)
  Register7/1 -> phase_rotate/4(im2_in)
  BitBasher1/1 -> AddSub/1
  ph_switch/1 -> AddSub/2
